simulink model "model"  (R2015b)
settings: Solver=VariableStepAuto  StartTime=0.0  StopTime=20.0  RelTol=1e-3
settings Model: Creator=yuji  LastModifiedBy=yuji

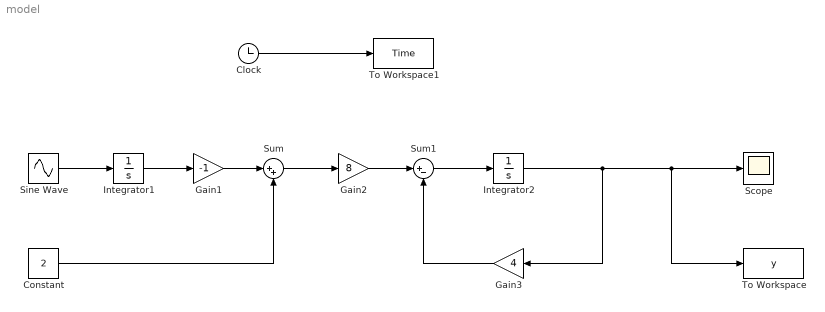
== system model ==
  Clock : Clock
  Constant : Constant  Value=2
  Gain1 : Gain  Gain=-1
  Gain2 : Gain  Gain=8
  Gain3 : Gain  Gain=4
  Integrator1 : Integrator  InitialCondition=-1
  Integrator2 : Integrator  InitialCondition=-5
  Scope : Scope
  Sine Wave : Sin  SampleTime=0.01
  Sum : Sum  Inputs=|++
  Sum1 : Sum  Inputs=|+-
  To Workspace : ToWorkspace  VariableName=y  SampleTime=-1
  To Workspace1 : ToWorkspace  VariableName=Time  SampleTime=-1
  wires:
  Clock/1 -> To Workspace1/1
  Integrator2/1 -> Scope/1, To Workspace/1, Gain3/1
  Gain3/1 -> Sum1/2
  Sum1/1 -> Integrator2/1
  Gain2/1 -> Sum1/1
  Sum/1 -> Gain2/1
  Gain1/1 -> Sum/1
  Sine Wave/1 -> Integrator1/1
  Integrator1/1 -> Gain1/1
  Constant/1 -> Sum/2
